simulink library "mbdriLib"  (R2021b)
settings: Solver=ode45  StartTime=0.0  StopTime=10.0  RelTol=1e-3  EnableMultiTasking=on
undefined symbols (not defined in the file or in its folder): ap, deg, DiscIntNeverNeededParam, Earth, env, flat2lla, Newton, rad, Raphson, s, uavData, WGS84, Xpoints, Ypoints, Zpoints
libraries: simulink x23, $bdroot x7, aerolibconvert2 x2, slpidlib x1, sharedtransform x1, SignalEditorBlockLib x1, aerolibtransform2 x1
(part 1 of 2)
settings Model: Creator=mlizarra  LastModifiedBy=promero
settings SolverCC: AlgebraicLoopSolver=TrustRegion
settings DataIOCC: LimitDataPoints=on
settings OptimizationCC: LifeSpan=inf
settings DebuggingCC: AllowSymbolicDim=off  SFUnexpectedBacktrackingDiag=warning  SFNoUnconditionalDefaultTransitionDiag=warning  SFExecutionAtInitializationDiag=none  SFMachineParentedDataDiag=warning  ArithmeticOperatorsInVariantConditions=warning
settings SFSimCC: SimUseLocalCustomCode=off  CustomCodeUndefinedFunction=UseInterfaceOnly
settings RTWCC: RTWUseLocalCustomCode=off
settings CodeAppCC: StateflowObjectComments=on
settings GRTTargetCC: TargetLangStandard=C89/C90 (ANSI)
settings ConfigComp: CovMetricSettings=dw  CovSaveCumulativeToWorkspaceVar=on  CovSaveSingleToWorkspaceVar=on  CovExternalEMLEnable=off

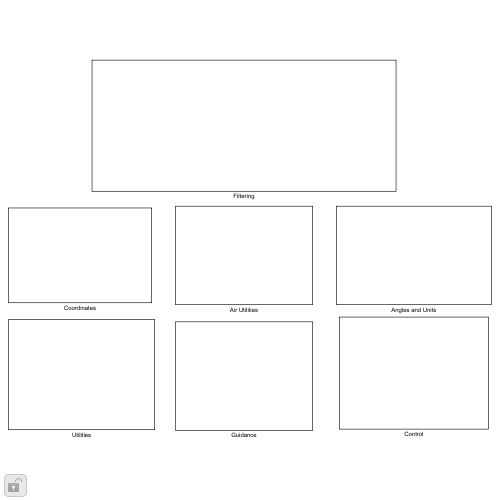
[thumbnail: Simulink's stored preview of the top-level diagram]
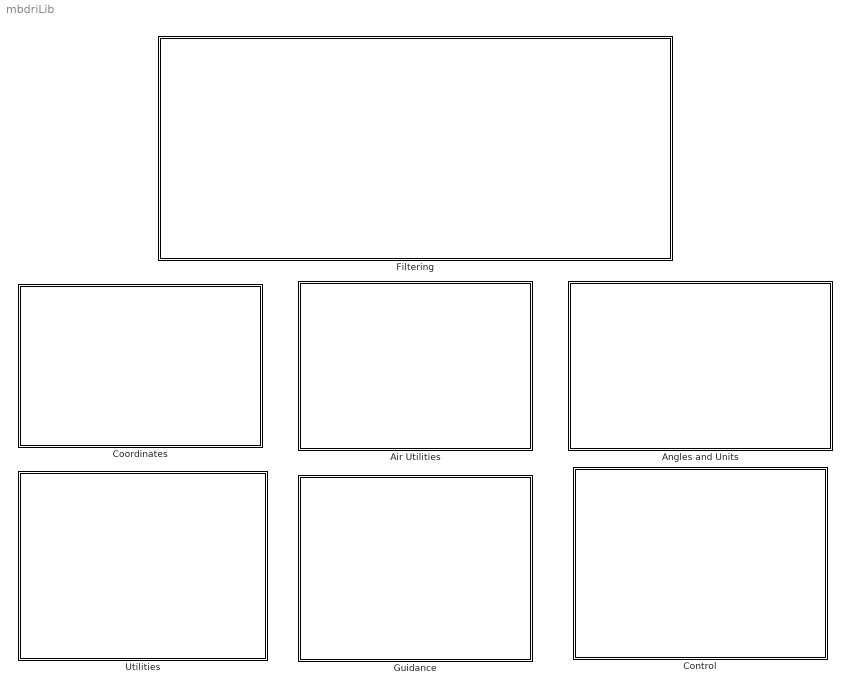
== system mbdriLib ==
  Air Utilities : Subsystem
  Angles and Units : Subsystem
  Control : Subsystem
  Coordinates : Subsystem
  Filtering : Subsystem
  Guidance : Subsystem
  Utilities : Subsystem

== system mbdriLib/Air Utilities ==
  Compute Airspeed : Subsystem

== system mbdriLib/Angles and Units ==
  Lateral Accel to Bank Angle : Subsystem
  psi_dot to phi : Subsystem

== system mbdriLib/Control ==
  PID Controller : Subsystem  mask(PID){Tsample=0.01, Ndelay=5, upperSaturationLimit=100, lowerSaturationLimit=-100}
      mask prompts: Tsample "Sample Time"; Ndelay "Integer delays for de/dt"; upperSaturationLimit "Upper Saturation Limit"; lowerSaturationLimit "Lower Saturation Limit"
      mask help: PID controller block with anti-windup and saturation limits. Implemented as a discrete forwardl integration which stops integrating when the output is saturated. Derivative is implemented as a numerical derivative with N integer delays to smooth output.
      mask Display:
      | disp('PID')
      | port_label('input',1,'error')
      | port_label('input',3,'gains')
      | port_label('input',2,'reset')
      | port_label('output',1,'output')

== system mbdriLib/Coordinates ==
  RL2B : Subsystem

== system mbdriLib/Filtering ==
  1D Discrete Filter : Subsystem  RTWFcnName=TustinFilter3D  mask{bw=40, TSample=0.01}
      mask prompts: bw "Bandwith (Hz)"; TSample "Sample Time"
      mask init:
      | tau = 1/(2*pi*bw);
      | zval = [];
      | pval = -1/tau;
      | kval = 1/tau;
      | 
      | set_param(gcb,'AttributesFormatString', ['Fc = ' num2str(bw)]);
      settings: AttributesFormatString=Fc = 40  RTWFcnNameOpts=User specified  RTWFileNameOpts=Use function name
      mask Display:
      | droots(zval,pval,kval)
      | port_label('input',1,'1D')
  3D Discrete Filter : Subsystem  RTWFcnName=TustinFilter3D  mask{bw=40, TSample=0.01}
      mask prompts: bw "Bandwith (Hz)"; TSample "Sample Time"
      mask init:
      | tau = 1/(2*pi*bw);
      | zval = [];
      | pval = -1/tau;
      | kval = 1/tau;
      | 
      | set_param(gcb,'AttributesFormatString', ['Fc = ' num2str(bw)]);
      settings: AttributesFormatString=Fc = 40  RTWFcnNameOpts=User specified  RTWFileNameOpts=Use function name
      mask Display:
      | droots(zval,pval,kval)
      | port_label('input',1,'3D')
  Complementary Filter : Subsystem  mask{omega=20, T=0.01}
      mask prompts: omega "Cutoff Freq (rad/sec)"; T "Sample Time"
  RateAid for GPS : MATLAB Function  TreatAsAtomicUnit=on
  ZPK 1D Discrete Filter : Subsystem  RTWFcnName=TustinFilter3D  mask{zval=[], pval=[0], kval=1, TSample=0.01}
      mask prompts: zval "Zeros"; pval "Poles"; kval "Gains"; TSample "Sample Time"
      settings: RTWFcnNameOpts=User specified  RTWFileNameOpts=Use function name
      mask Display:
      | droots(zval,pval,kval)
      | port_label('input',1,'1D')
  ZPK 3D Filter : Subsystem  RTWFcnName=TustinFilter3D  mask{zval=[], pval=-1/20, kval=1, TSample=0.01}
      mask prompts: zval "Zeros"; pval "Poles"; kval "Gains"; TSample "Sample Time"
      settings: RTWFcnNameOpts=User specified  RTWFileNameOpts=Use function name
      mask Display:
      | droots(zval,pval,kval)
      | port_label('input',1,'3D')

== system mbdriLib/Guidance ==
  L2+ Guidance Law : Subsystem
  Wp Switching Logic : Stateflow chart  TreatAsAtomicUnit=on

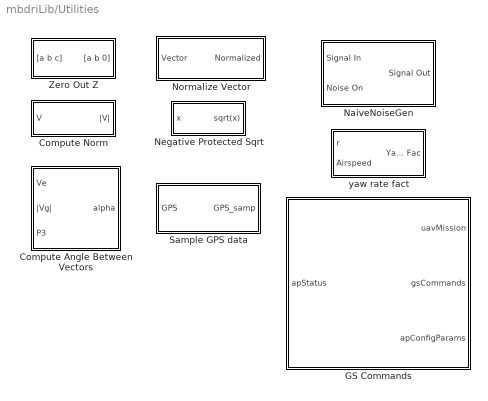
== system mbdriLib/Utilities ==
  " Compute Norm" : Subsystem
  Compute Angle Between Vectors : Subsystem
  "GS Commands " : Subsystem  Variant=on
  NaiveNoiseGen : Subsystem  mask{np=[0.0005], st=ap.apSampleTime, ng=0.2, ns=[1387]}
      mask prompts: np "Noise Power"; st "Sample Time"; ng "Noise Gain"; ns "Noise Seed"
  Negative Protected Sqrt : Subsystem
  Normalize Vector : Subsystem
  Sample GPS data : Subsystem
  Zero Out Z : Subsystem
  yaw rate fact : Subsystem

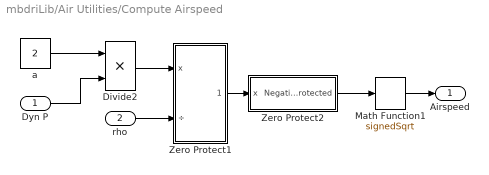
== system mbdriLib/Air Utilities/Compute Airspeed ==
  Dyn P : Inport  Unit=Pa
  rho : Inport  Port=2  Unit=kg/m^3
  Divide2 : Product
  Math Function1 : Sqrt  Operator=signedSqrt  AlgorithmType=Newton-Raphson  SaturateOnIntegerOverflow=on
  Zero Protect1 : Subsystem
      mask Display:
      | disp('Zero\n Protected\nDivision')
      | port_label('input',1,'x')
      | port_label('input',2,'÷')
  Zero Protect2 : Subsystem
      mask Display:
      | disp('Negative\n Protection')
      | port_label('input',1,'u')
      | port_label('output',1,'y')
  a : Constant  Value=2
      settings: AttributesFormatString=%<Value>
  "Airspeed " : Outport  Unit=m/s  VectorParamsAs1DForOutWhenUnconnected=off
  wires:
  Dyn P/1 -> Divide2/2
  a/1 -> Divide2/1
  Zero Protect2/1(Negative Protected) -> Math Function1/1
  Math Function1/1 -> "Airspeed "/1
  Divide2/1 -> Zero Protect1/1(x)
  rho/1 -> Zero Protect1/2(÷)
  Zero Protect1/1(Zero Protected) -> Zero Protect2/1(x)

== system mbdriLib/Angles and Units/Lateral Accel to Bank Angle ==
  a_c : Inport
  Constant : Constant  Value=env.ISA_g
      settings: AttributesFormatString=%<Value>
  Product : Product  Inputs=*/  RndMeth=Zero
  Trigonometric Function : Trigonometry  Operator=atan
  phi_c : Outport  VectorParamsAs1DForOutWhenUnconnected=off
  wires:
  Trigonometric Function/1 -> phi_c/1
  Product/1 -> Trigonometric Function/1
  Constant/1 -> Product/2
  a_c/1 -> Product/1

== system mbdriLib/Angles and Units/psi_dot to phi ==
  psi_dot : Inport  Unit=rad/sec
  U_m : Inport  Port=2  Unit=m/s
  Constant1 : Constant  Value=env.ISA_g
      settings: AttributesFormatString=%<Value>
  Divide : Product  Inputs=**/
  Trigonometric Function : Trigonometry  Operator=atan
  phi : Outport  Unit=rad  VectorParamsAs1DForOutWhenUnconnected=off
  wires:
  psi_dot/1 -> Divide/1
  U_m/1 -> Divide/2
  Constant1/1 -> Divide/3
  Trigonometric Function/1 -> phi/1
  Divide/1 -> Trigonometric Function/1

== system mbdriLib/Control/PID Controller ==
  Error : Inport
  Reset : Inport  Port=2
  PIDGains : Inport  Port=3
  Cast To Boolean : DataTypeConversion  OutDataTypeStr=boolean
  Demux : Demux  Outputs=3
  PID Controller : slpidlib/PID Controller  Controller=PID  Form=Parallel  TimeDomain=Discrete-time  UseExternalTs=off  SampleTime=Tsample  IntegratorMethod=Trapezoidal  FilterMethod=Forward Euler  ControllerParametersSource=external  P=1  I=1  D=0  UseFilter=on  N=100  TunerSelectOption=Transfer Function Based (PID Tuner App)  InitialConditionSource=internal  InitialConditionForIntegrator=0  InitialConditionForFilter=0  DifferentiatorICPrevScaledInput=0  ExternalReset=level  TrackingMode=off  Kt=1  LimitOutput=on  SatLimitsSource=internal  UpperSaturationLimit=upperSaturationLimit  LowerSaturationLimit=lowerSaturationLimit  LinearizeAsGain=on  AntiWindupMode=clamping  Kb=1  POutMin=[]  POutMax=[]  IOutMin=[]  IOutMax=[]  DOutMin=[]  DOutMax=[]  NOutMin=[]  NOutMax=[]  SumOutMin=[]  SumOutMax=[]  SaturationOutMin=[]  SaturationOutMax=[]  PParamMin=[]  PParamMax=[]  IParamMin=[]  IParamMax=[]  DParamMin=[]  DParamMax=[]  NParamMin=[]  NParamMax=[]  KbParamMin=[]  KbParamMax=[]  KtParamMin=[]  KtParamMax=[]  KbOutMin=[]  KbOutMax=[]  KtOutMin=[]  KtOutMax=[]  IntegratorOutMin=[]  IntegratorOutMax=[]  FilterOutMin=[]  FilterOutMax=[]  SumI1OutMin=[]  SumI1OutMax=[]  SumI2OutMin=[]  SumI2OutMax=[]  SumI3OutMin=[]  SumI3OutMax=[]  SumI4OutMin=[]  SumI4OutMax=[]  SumDOutMin=[]  SumDOutMax=[]  DifferentiatorOutMin=[]  DifferentiatorOutMax=[]  FilterDiffOutCoefMin=[]  FilterDiffOutCoefMax=[]  ReciprocalOutMin=[]  ReciprocalOutMax=[]  SumDenOutMin=[]  SumDenOutMax=[]  SumNumOutMin=[]  SumNumOutMax=[]  DivideOutMin=[]  DivideOutMax=[]  UdiffTsProdOutMin=[]  UdiffTsProdOutMax=[]  NTsProdOutMin=[]  NTsProdOutMax=[]  UintegralTsProdOutMin=[]  UintegralTsProdOutMax=[]  UngainTsProdOutMin=[]  UngainTsProdOutMax=[]  IntegratorContinuousStateAttributes=''  IntegratorStateMustResolveToSignalObject=off  IntegratorRTWStateStorageClass=Auto  FilterContinuousStateAttributes=''  FilterStateMustResolveToSignalObject=off  FilterRTWStateStorageClass=Auto  ParallelPVariant=ExternalParameters  IdealPVariant=Disabled  IVariant=ExternalParameters  DVariant=ExternalParameters  IntegratorVariant=Discrete  SatVariant=Enabled  AWVariant=DiscClampingParallel  PCopyVariant=Disabled  TRVariant=Disabled  FdbkBlocksVariant=Feedback  IdealPFdbkVariant=Passthrough  SatFdbkVariant=Passthrough  DerivativeFilterVariant=ForwardEulerFilter  NVariant=ExternalParameters  NCopyVariant=Disabled  FilterICVariant=InternalICsFilter  IntegratorICVariant=InternalICs  ExternalResetVariant=ExternalReset  TRSumVariant=Passthrough  SumFdbkVariant=Enabled  SumVariant=Sum_PID  TsampFilterVariant=InternalTs  TsampNgainVariant=Passthrough  TsampIntegralVariant=Passthrough  ExternalSaturationOutDataTypeStr=Inherit: Same as second input
  delayTime1 : Constant  Value=Ndelay
      settings: AttributesFormatString=%<Value>
  Output : Outport  VectorParamsAs1DForOutWhenUnconnected=off
  wires:
  PIDGains/1 -> Demux/1
  Demux/1 -> PID Controller/2
  Demux/2 -> PID Controller/3
  Demux/3 -> PID Controller/4
  delayTime1/1 -> PID Controller/5
  Reset/1 -> Cast To Boolean/1
  PID Controller/1 -> Output/1
  Error/1 -> PID Controller/1
  Cast To Boolean/1 -> PID Controller/6

== system mbdriLib/Coordinates/RL2B ==
  Euler : Inport
  Rotation Angles to Direction Cosine Matrix : sharedtransform/Rotation Angles to Direction Cosine Matrix  rotationOrder=ZYX  aMode=aMode
      settings: SourceProductBaseCode=AE,PW,DR,MT,UV,VE
  Selector : Selector  InputPortWidth=3  IndexOptions=Index vector (dialog)  Indices=[3 2 1]  OutputSizes=1
  RL2B : Outport  VectorParamsAs1DForOutWhenUnconnected=off
  wires:
  Selector/1 -> Rotation Angles to Direction Cosine Matrix/1
  Euler/1 -> Selector/1
  Rotation Angles to Direction Cosine Matrix/1 -> RL2B/1

== system mbdriLib/Filtering/1D Discrete Filter ==
  In1 : Inport
  Filter4 : Subsystem  mask{Zeros=zval, Poles=pval, Gain=kval, AbsTol=auto, SampleTime=TSample, method=tustin, Wc=1}
      mask prompts: Zeros "Zeros (enter in s-main:)"; Poles "Poles (enter in s-domain:)"; Gain "Gain (enter in s-domain:)"; AbsTol "Absolute tolerance:"; SampleTime "Sample time:"; Wc "Critical Frequency (Hz):"
      mask init:
      | H = zpk(Zeros, Poles, Gain);
      | Hd = c2d(H, SampleTime, 'tustin');
      | [z, p, g] = zpkdata(Hd);
      | z_d = z{:};
      | p_d = p{:};
      | g_d = g;
      mask TypeOptions method: zoh | foh | tustin | prewarp | matched
      mask Display: droots(Zeros,Poles,Gain)
  Out1 : Outport  VectorParamsAs1DForOutWhenUnconnected=off
  wires:
  Filter4/1(Out1) -> Out1/1
  In1/1 -> Filter4/1(In1)

== system mbdriLib/Filtering/3D Discrete Filter ==
  In1 : Inport
  Demux : Demux  Outputs=3
  Filter1 : Subsystem  mask{Zeros=zval, Poles=pval, Gain=kval, AbsTol=auto, SampleTime=TSample, method=tustin, Wc=1}
      mask prompts: Zeros "Zeros (enter in s-main:)"; Poles "Poles (enter in s-domain:)"; Gain "Gain (enter in s-domain:)"; AbsTol "Absolute tolerance:"; SampleTime "Sample time:"; Wc "Critical Frequency (Hz):"
      mask init:
      | H = zpk(Zeros, Poles, Gain);
      | Hd = c2d(H, SampleTime, 'tustin');
      | [z, p, g] = zpkdata(Hd);
      | z_d = z{:};
      | p_d = p{:};
      | g_d = g;
      mask TypeOptions method: zoh | foh | tustin | prewarp | matched
      mask Display: droots(Zeros,Poles,Gain)
  Filter2 : Subsystem  mask{Zeros=zval, Poles=pval, Gain=kval, AbsTol=auto, SampleTime=TSample, method=tustin, Wc=1}
      mask prompts: Zeros "Zeros (enter in s-main:)"; Poles "Poles (enter in s-domain:)"; Gain "Gain (enter in s-domain:)"; AbsTol "Absolute tolerance:"; SampleTime "Sample time:"; Wc "Critical Frequency (Hz):"
      mask init:
      | H = zpk(Zeros, Poles, Gain);
      | Hd = c2d(H, SampleTime, 'tustin');
      | [z, p, g] = zpkdata(Hd);
      | z_d = z{:};
      | p_d = p{:};
      | g_d = g;
      mask TypeOptions method: zoh | foh | tustin | prewarp | matched
      mask Display: droots(Zeros,Poles,Gain)
  Filter4 : Subsystem  mask{Zeros=zval, Poles=pval, Gain=kval, AbsTol=auto, SampleTime=TSample, method=tustin, Wc=1}
      mask prompts: Zeros "Zeros (enter in s-main:)"; Poles "Poles (enter in s-domain:)"; Gain "Gain (enter in s-domain:)"; AbsTol "Absolute tolerance:"; SampleTime "Sample time:"; Wc "Critical Frequency (Hz):"
      mask init:
      | H = zpk(Zeros, Poles, Gain);
      | Hd = c2d(H, SampleTime, 'tustin');
      | [z, p, g] = zpkdata(Hd);
      | z_d = z{:};
      | p_d = p{:};
      | g_d = g;
      mask TypeOptions method: zoh | foh | tustin | prewarp | matched
      mask Display: droots(Zeros,Poles,Gain)
  Mux : Mux  Inputs=3
  Out1 : Outport  VectorParamsAs1DForOutWhenUnconnected=off
  wires:
  Filter2/1(Out1) -> Mux/3
  Filter1/1(Out1) -> Mux/2
  Filter4/1(Out1) -> Mux/1
  Demux/3 -> Filter2/1(In1)
  Demux/2 -> Filter1/1(In1)
  Demux/1 -> Filter4/1(In1)
  In1/1 -> Demux/1
  Mux/1 -> Out1/1

== system mbdriLib/Filtering/Complementary Filter ==
  Rate : Inport
  LoPass : Inport  Port=2
  CutOff : Gain  Gain=omega
      settings: AttributesFormatString=%<Gain>
  Sum : Sum  Inputs=++|
  Sum1 : Sum  Inputs=|+-
  Unit Delay : UnitDelay  SampleTime=ap.apSampleTime  HasFrameUpgradeWarning=on
  ZPK 1D Discrete Filter : $bdroot/Filtering/ZPK 1D Discrete Filter  zval=[]  pval=[0]  kval=1  TSample=ap.apSampleTime
  Blend : Outport  VectorParamsAs1DForOutWhenUnconnected=off
  wires:
  ZPK 1D Discrete Filter/1 -> Blend/1, Unit Delay/1
  Sum/1 -> ZPK 1D Discrete Filter/1  "rate_hat"
  Rate/1 -> Sum/1
  CutOff/1 -> Sum/2
  Sum1/1 -> CutOff/1
  LoPass/1 -> Sum1/1
  Unit Delay/1 -> Sum1/2

== system mbdriLib/Filtering/ZPK 1D Discrete Filter ==
  In1 : Inport
  Filter2 : Subsystem  mask{Zeros=zval, Poles=pval, Gain=kval, AbsTol=auto, SampleTime=TSample, method=tustin, Wc=1}
      mask prompts: Zeros "Zeros (enter in s-main:)"; Poles "Poles (enter in s-domain:)"; Gain "Gain (enter in s-domain:)"; AbsTol "Absolute tolerance:"; SampleTime "Sample time:"; Wc "Critical Frequency (Hz):"
      mask init:
      | H = zpk(Zeros, Poles, Gain);
      | Hd = c2d(H, SampleTime, 'tustin');
      | [z, p, g] = zpkdata(Hd);
      | z_d = z{:};
      | p_d = p{:};
      | g_d = g;
      mask TypeOptions method: zoh | foh | tustin | prewarp | matched
      mask Display: droots(Zeros,Poles,Gain)
  Out1 : Outport  VectorParamsAs1DForOutWhenUnconnected=off
  wires:
  In1/1 -> Filter2/1(In1)
  Filter2/1(Out1) -> Out1/1

== system mbdriLib/Filtering/ZPK 3D Filter ==
  In1 : Inport
  Demux : Demux  Outputs=3
  Filter1 : Subsystem  mask{Zeros=zval, Poles=pval, Gain=kval, AbsTol=auto, SampleTime=TSample, method=tustin, Wc=1}
      mask prompts: Zeros "Zeros (enter in s-main:)"; Poles "Poles (enter in s-domain:)"; Gain "Gain (enter in s-domain:)"; AbsTol "Absolute tolerance:"; SampleTime "Sample time:"; Wc "Critical Frequency (Hz):"
      mask init:
      | H = zpk(Zeros, Poles, Gain);
      | Hd = c2d(H, SampleTime, 'tustin');
      | [z, p, g] = zpkdata(Hd);
      | z_d = z{:};
      | p_d = p{:};
      | g_d = g;
      mask TypeOptions method: zoh | foh | tustin | prewarp | matched
      mask Display: droots(Zeros,Poles,Gain)
  Filter2 : Subsystem  mask{Zeros=zval, Poles=pval, Gain=kval, AbsTol=auto, SampleTime=TSample, method=tustin, Wc=1}
      mask prompts: Zeros "Zeros (enter in s-main:)"; Poles "Poles (enter in s-domain:)"; Gain "Gain (enter in s-domain:)"; AbsTol "Absolute tolerance:"; SampleTime "Sample time:"; Wc "Critical Frequency (Hz):"
      mask init:
      | H = zpk(Zeros, Poles, Gain);
      | Hd = c2d(H, SampleTime, 'tustin');
      | [z, p, g] = zpkdata(Hd);
      | z_d = z{:};
      | p_d = p{:};
      | g_d = g;
      mask TypeOptions method: zoh | foh | tustin | prewarp | matched
      mask Display: droots(Zeros,Poles,Gain)
  Filter4 : Subsystem  mask{Zeros=zval, Poles=pval, Gain=kval, AbsTol=auto, SampleTime=TSample, method=tustin, Wc=1}
      mask prompts: Zeros "Zeros (enter in s-main:)"; Poles "Poles (enter in s-domain:)"; Gain "Gain (enter in s-domain:)"; AbsTol "Absolute tolerance:"; SampleTime "Sample time:"; Wc "Critical Frequency (Hz):"
      mask init:
      | H = zpk(Zeros, Poles, Gain);
      | Hd = c2d(H, SampleTime, 'tustin');
      | [z, p, g] = zpkdata(Hd);
      | z_d = z{:};
      | p_d = p{:};
      | g_d = g;
      mask TypeOptions method: zoh | foh | tustin | prewarp | matched
      mask Display: droots(Zeros,Poles,Gain)
  Mux : Mux  Inputs=3
  Out1 : Outport  VectorParamsAs1DForOutWhenUnconnected=off
  wires:
  Mux/1 -> Out1/1
  In1/1 -> Demux/1
  Demux/1 -> Filter4/1(In1)
  Demux/2 -> Filter1/1(In1)
  Demux/3 -> Filter2/1(In1)
  Filter4/1(Out1) -> Mux/1
  Filter1/1(Out1) -> Mux/2
  Filter2/1(Out1) -> Mux/3

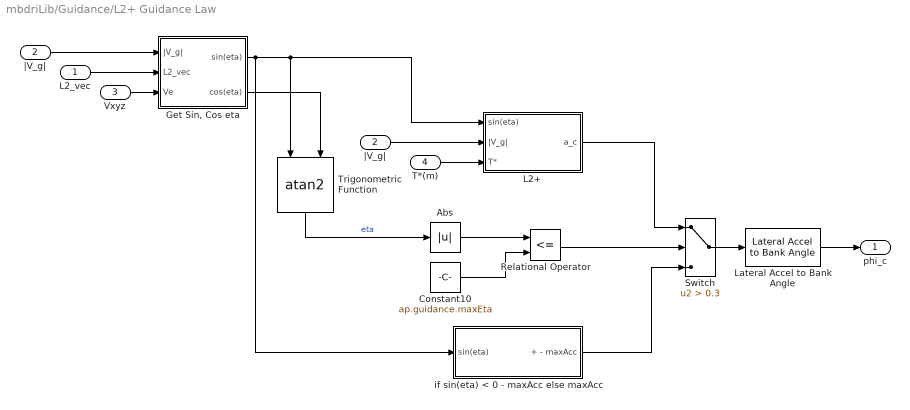
== system mbdriLib/Guidance/L2+ Guidance Law ==
  L2_vec : Inport
  |V_g| : Inport  Port=2  Unit=m/s
  Vxyz : Inport  Port=3  Unit=m/s
  T*(m) : Inport  Port=4  Unit=m
  Abs : Abs
  Constant10 : Constant  Value=ap.guidance.maxEta
      settings: AttributesFormatString=%<Value>
  "Get Sin, Cos eta" : Subsystem
  L2+ : Subsystem
  Lateral Accel to Bank Angle : $bdroot/Angles and Units/Lateral Accel to  Bank Angle  SystemSampleTime=-1  VariantActivationTime=update diagram  Latency=0  AutoFrameSizeCalculation=off
  Relational Operator : RelationalOperator  Operator=<=  OutDataTypeStr=boolean  RndMeth=Nearest
  Switch : Switch  Criteria=u2 > Threshold  Threshold=0.3
  Trigonometric Function : Trigonometry  Operator=atan2
  "if sin(eta) < 0 - maxAcc else maxAcc " : Subsystem
  "|V_g| " : InportShadow  Port=2  Unit=m/s
  phi_c : Outport  Unit=rad  VectorParamsAs1DForOutWhenUnconnected=off
  wires:
  "Get Sin, Cos eta"/2(cos(eta)) -> Trigonometric Function/2
  L2+/1(a_c) -> Switch/1
  Lateral Accel to Bank Angle/1 -> phi_c/1
  T*(m)/1 -> L2+/3(T*)
  "|V_g| "/1 -> L2+/2(|V_g|)
  "Get Sin, Cos eta"/1(sin(eta)) -> Trigonometric Function/1, L2+/1(sin(eta)), "if sin(eta) < 0 - maxAcc else maxAcc "/1(sin(eta))
  Trigonometric Function/1 -> Abs/1  "eta"
  Abs/1 -> Relational Operator/1
  Constant10/1 -> Relational Operator/2
  Relational Operator/1 -> Switch/2
  "if sin(eta) < 0 - maxAcc else maxAcc "/1(+ - maxAcc) -> Switch/3
  Switch/1 -> Lateral Accel to Bank Angle/1
  |V_g|/1 -> "Get Sin, Cos eta"/1(|V_g|)
  L2_vec/1 -> "Get Sin, Cos eta"/2(L2_vec)
  Vxyz/1 -> "Get Sin, Cos eta"/3(Ve)

== system mbdriLib/Utilities/ Compute Norm ==
  V : Inport
  Dot Product : DotProduct  InputSameDT=on  OutDataTypeStr=Inherit: Inherit via internal rule
  Negative Protected Sqrt : $bdroot/Utilities/Negative Protected Sqrt  SystemSampleTime=-1  VariantActivationTime=update diagram  Latency=0  AutoFrameSizeCalculation=off
  |V| : Outport  VectorParamsAs1DForOutWhenUnconnected=off
  wires:
  Dot Product/1 -> Negative Protected Sqrt/1
  V/1 -> Dot Product/1, Dot Product/2
  Negative Protected Sqrt/1 -> |V|/1

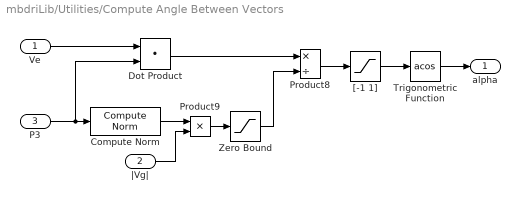
== system mbdriLib/Utilities/Compute Angle Between Vectors ==
  Ve : Inport
  |Vg| : Inport  Port=2
  P3 : Inport  Port=3
  " Compute Norm" : $bdroot/Utilities/ Compute Norm  SystemSampleTime=-1  VariantActivationTime=update diagram  Latency=0  AutoFrameSizeCalculation=off
  Dot Product : DotProduct  InputSameDT=on  OutDataTypeStr=Inherit: Inherit via internal rule
  Product8 : Product  Inputs=*/  RndMeth=Zero
  Product9 : Product  RndMeth=Zero
  Trigonometric Function : Trigonometry  Operator=acos
  Zero Bound : Saturate  UpperLimit=inf  LowerLimit=0.001
      settings: AttributesFormatString="[%<LowerLimit>  %<UpperLimit>]"
  "[-1 1]" : Saturate  UpperLimit=1  LowerLimit=-1
      settings: AttributesFormatString="[%<LowerLimit>  %<UpperLimit>]"
  alpha : Outport  VectorParamsAs1DForOutWhenUnconnected=off
  wires:
  P3/1 -> " Compute Norm"/1, Dot Product/2
  Ve/1 -> Dot Product/1
  Dot Product/1 -> Product8/1
  " Compute Norm"/1 -> Product9/1
  |Vg|/1 -> Product9/2
  Product9/1 -> Zero Bound/1
  Product8/1 -> "[-1 1]"/1
  "[-1 1]"/1 -> Trigonometric Function/1
  Zero Bound/1 -> Product8/2
  Trigonometric Function/1 -> alpha/1

== system mbdriLib/Utilities/GS Commands  ==
  apStatus : Inport  OutDataTypeStr=Bus: apStatusBus
  Use QGroundControl : Subsystem  VariantControl=useQGCvar
  Use Simulink : Subsystem  VariantControl=useSLvar
  uavMission : Outport  OutDataTypeStr=Bus: waypoint  VectorParamsAs1DForOutWhenUnconnected=off
  gsCommands : Outport  Port=2  OutDataTypeStr=Bus: gsCommandsBus  VectorParamsAs1DForOutWhenUnconnected=off
  apConfigParams : Outport  Port=3  OutDataTypeStr=Bus: apConfigParamsBus  VectorParamsAs1DForOutWhenUnconnected=off

== system mbdriLib/Utilities/NaiveNoiseGen ==
  Signal In : Inport
  Noise On : Inport  Port=2
  Add : Sum
  Band-Limited White Noise : simulink/Sources/Band-Limited White Noise  Cov=np  Ts=st  seed=ns
  Gain : Gain  Gain=ng
      settings: AttributesFormatString=%<Gain>
  Switch : Switch  Threshold=0.3
  Signal Out : Outport  VectorParamsAs1DForOutWhenUnconnected=off
  wires:
  Band-Limited White Noise/1 -> Gain/1
  Add/1 -> Switch/1
  Noise On/1 -> Switch/2
  Switch/1 -> Signal Out/1
  Signal In/1 -> Switch/3, Add/1
  Gain/1 -> Add/2

== system mbdriLib/Utilities/Negative Protected Sqrt ==
  x : Inport
  Math Function1 : Sqrt  OutputSignalType=real  AlgorithmType=Newton-Raphson  SaturateOnIntegerOverflow=on
      settings: AttributesFormatString=%<AlgorithmType>
  Zero Bound : Saturate  UpperLimit=inf  LowerLimit=0.001
      settings: AttributesFormatString="[%<LowerLimit>  %<UpperLimit>]"
  sqrt(x) : Outport  VectorParamsAs1DForOutWhenUnconnected=off
  wires:
  x/1 -> Zero Bound/1
  Math Function1/1 -> sqrt(x)/1
  Zero Bound/1 -> Math Function1/1

== system mbdriLib/Utilities/Normalize Vector ==
  Vector : Inport
  " Compute Norm" : $bdroot/Utilities/ Compute Norm  SystemSampleTime=-1  VariantActivationTime=update diagram  Latency=0  AutoFrameSizeCalculation=off
  Divide : Product  Inputs=*/
  Normalized : Outport  VectorParamsAs1DForOutWhenUnconnected=off
  wires:
  Vector/1 -> Divide/1, " Compute Norm"/1
  " Compute Norm"/1 -> Divide/2
  Divide/1 -> Normalized/1

== system mbdriLib/Utilities/Sample GPS data ==
  GPS : Inport
  Rate Transition : RateTransition  Deterministic=off  OutPortSampleTime=sensors.gpsRefreshRate
      settings: AttributesFormatString=%<OutPortSampleTime>
  GPS_samp : Outport  VectorParamsAs1DForOutWhenUnconnected=off
  wires:
  GPS/1 -> Rate Transition/1
  Rate Transition/1 -> GPS_samp/1

== system mbdriLib/Utilities/Zero Out Z ==
  "[a b c]" : Inport
  Constant : Constant  Value=0
      settings: AttributesFormatString=%<Value>
  Demux : Demux  Outputs=[2 1]
  Mux : Mux  Inputs=2
  Terminator : Terminator
  "[a b 0]" : Outport  VectorParamsAs1DForOutWhenUnconnected=off
  wires:
  "[a b c]"/1 -> Demux/1
  Constant/1 -> Mux/2
  Demux/2 -> Terminator/1
  Mux/1 -> "[a b 0]"/1
  Demux/1 -> Mux/1

== system mbdriLib/Utilities/yaw rate fact ==
  r : Inport
  Airspeed : Inport  Port=2
  Cmq3 : Constant  Value=.5
      settings: AttributesFormatString=%<Value>
  Cmq4 : Constant  Value=uavData.geometry.span
      settings: AttributesFormatString=%<Value>
  Product1 : Product  Inputs=***/  SaturateOnIntegerOverflow=on  OutDataTypeStr=Inherit: Same as first input
  Saturation : Saturate  UpperLimit=inf  LowerLimit=0.1
      settings: AttributesFormatString="[%<LowerLimit>  %<UpperLimit>]"
  Yaw Rate Fac : Outport  VectorParamsAs1DForOutWhenUnconnected=off
  wires:
  Saturation/1 -> Product1/4
  Airspeed/1 -> Saturation/1
  Cmq4/1 -> Product1/3
  Cmq3/1 -> Product1/2
  r/1 -> Product1/1
  Product1/1 -> Yaw Rate Fac/1

== system mbdriLib/Air Utilities/Compute Airspeed/Zero Protect1 ==
  x : Inport
  ÷ : Inport  Port=2
  Divide2 : Product  Inputs=*/
  Switch : Switch  Criteria=u2 ~= 0  Threshold=0.1  OutDataTypeStr=Inherit: Inherit via back propagation
  Zero Value : Constant  Value=0
  Zero Protected : Outport  VectorParamsAs1DForOutWhenUnconnected=off
  wires:
  ÷/1 -> Switch/2, Divide2/2
  Zero Value/1 -> Switch/3
  Switch/1 -> Zero Protected/1
  Divide2/1 -> Switch/1
  x/1 -> Divide2/1

== system mbdriLib/Air Utilities/Compute Airspeed/Zero Protect2 ==
  x : Inport
  Switch : Switch  OutDataTypeStr=Inherit: Inherit via back propagation
  Zero Value : Constant  Value=0
  Negative Protected : Outport  VectorParamsAs1DForOutWhenUnconnected=off
  wires:
  x/1 -> Switch/2, Switch/1
  Switch/1 -> Negative Protected/1
  Zero Value/1 -> Switch/3

== system mbdriLib/Filtering/1D Discrete Filter/Filter4 ==
  In1 : Inport
  Discrete Zero-Pole : DiscreteZeroPole  Zeros=z_d  Poles=p_d  Gain=g_d  SampleTime=-1
  Out1 : Outport  VectorParamsAs1DForOutWhenUnconnected=off
  wires:
  Discrete Zero-Pole/1 -> Out1/1
  In1/1 -> Discrete Zero-Pole/1

== system mbdriLib/Filtering/3D Discrete Filter/Filter1 ==
  In1 : Inport
  Discrete Zero-Pole : DiscreteZeroPole  Zeros=z_d  Poles=p_d  Gain=g_d  SampleTime=-1
  Out1 : Outport  VectorParamsAs1DForOutWhenUnconnected=off
  wires:
  Discrete Zero-Pole/1 -> Out1/1
  In1/1 -> Discrete Zero-Pole/1

== system mbdriLib/Filtering/3D Discrete Filter/Filter2 ==
  In1 : Inport
  Discrete Zero-Pole : DiscreteZeroPole  Zeros=z_d  Poles=p_d  Gain=g_d  SampleTime=-1
  Out1 : Outport  VectorParamsAs1DForOutWhenUnconnected=off
  wires:
  In1/1 -> Discrete Zero-Pole/1
  Discrete Zero-Pole/1 -> Out1/1

== system mbdriLib/Filtering/3D Discrete Filter/Filter4 ==
  In1 : Inport
  Discrete Zero-Pole : DiscreteZeroPole  Zeros=z_d  Poles=p_d  Gain=g_d  SampleTime=-1
  Out1 : Outport  VectorParamsAs1DForOutWhenUnconnected=off
  wires:
  In1/1 -> Discrete Zero-Pole/1
  Discrete Zero-Pole/1 -> Out1/1

== system mbdriLib/Filtering/ZPK 1D Discrete Filter/Filter2 ==
  In1 : Inport
  Discrete Zero-Pole : DiscreteZeroPole  Zeros=z_d  Poles=p_d  Gain=g_d  SampleTime=-1
  Out1 : Outport  VectorParamsAs1DForOutWhenUnconnected=off
  wires:
  In1/1 -> Discrete Zero-Pole/1
  Discrete Zero-Pole/1 -> Out1/1

== system mbdriLib/Filtering/ZPK 3D Filter/Filter1 ==
  In1 : Inport
  Discrete Zero-Pole : DiscreteZeroPole  Zeros=z_d  Poles=p_d  Gain=g_d  SampleTime=-1
  Out1 : Outport  VectorParamsAs1DForOutWhenUnconnected=off
  wires:
  In1/1 -> Discrete Zero-Pole/1
  Discrete Zero-Pole/1 -> Out1/1

== system mbdriLib/Filtering/ZPK 3D Filter/Filter2 ==
  In1 : Inport
  Discrete Zero-Pole : DiscreteZeroPole  Zeros=z_d  Poles=p_d  Gain=g_d  SampleTime=-1
  Out1 : Outport  VectorParamsAs1DForOutWhenUnconnected=off
  wires:
  Discrete Zero-Pole/1 -> Out1/1
  In1/1 -> Discrete Zero-Pole/1

== system mbdriLib/Filtering/ZPK 3D Filter/Filter4 ==
  In1 : Inport
  Discrete Zero-Pole : DiscreteZeroPole  Zeros=z_d  Poles=p_d  Gain=g_d  SampleTime=-1
  Out1 : Outport  VectorParamsAs1DForOutWhenUnconnected=off
  wires:
  Discrete Zero-Pole/1 -> Out1/1
  In1/1 -> Discrete Zero-Pole/1

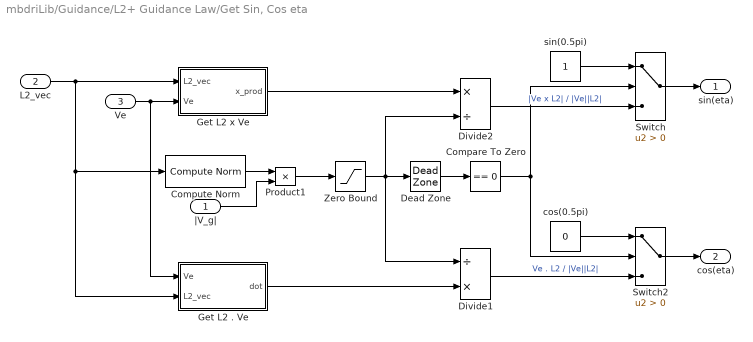
== system mbdriLib/Guidance/L2+ Guidance Law/Get Sin, Cos eta ==
  |V_g| : Inport
  L2_vec : Inport  Port=2
  Ve : Inport  Port=3
  " Compute Norm" : $bdroot/Utilities/ Compute Norm  SystemSampleTime=-1  VariantActivationTime=update diagram  Latency=0  AutoFrameSizeCalculation=off
  Compare To Zero : simulink/Logic and Bit Operations/Compare To Zero  relop===  OutDataTypeStr=boolean  ZeroCross=off
  Dead Zone : DeadZone  LowerValue=-0.1  UpperValue=0.1  SaturateOnIntegerOverflow=on
  Divide1 : Product  Inputs=/*
  Divide2 : Product  Inputs=*/
  Get L2 . Ve : Subsystem
  Get L2 x Ve : Subsystem
  Product1 : Product  RndMeth=Zero
  Switch : Switch  Criteria=u2 > Threshold  ZeroCross=off
  Switch2 : Switch  Criteria=u2 > Threshold  ZeroCross=off
  Zero Bound : Saturate  UpperLimit=inf  LowerLimit=0.001
      settings: AttributesFormatString="[%<LowerLimit>  %<UpperLimit>]"
  cos(0.5pi) : Constant  Value=0
      settings: AttributesFormatString=%<Value>
  sin(0.5pi) : Constant
      settings: AttributesFormatString=%<Value>
  sin(eta) : Outport  VectorParamsAs1DForOutWhenUnconnected=off
  cos(eta) : Outport  Port=2  VectorParamsAs1DForOutWhenUnconnected=off
  wires:
  Compare To Zero/1 -> Switch/2, Switch2/2
  Dead Zone/1 -> Compare To Zero/1
  L2_vec/1 -> Get L2 x Ve/1(L2_vec), Get L2 . Ve/2(L2_vec), " Compute Norm"/1
  Ve/1 -> Get L2 x Ve/2(Ve), Get L2 . Ve/1(Ve)
  " Compute Norm"/1 -> Product1/1
  |V_g|/1 -> Product1/2
  Product1/1 -> Zero Bound/1
  Get L2 . Ve/1(dot) -> Divide1/2
  sin(0.5pi)/1 -> Switch/1
  Switch2/1 -> cos(eta)/1
  cos(0.5pi)/1 -> Switch2/1
  Divide1/1 -> Switch2/3  "Ve . L2 / |Ve||L2|"
  Get L2 x Ve/1(x_prod) -> Divide2/1
  Divide2/1 -> Switch/3  "|Ve x L2| / |Ve||L2|"
  Switch/1 -> sin(eta)/1
  Zero Bound/1 -> Dead Zone/1, Divide2/2, Divide1/1

== system mbdriLib/Guidance/L2+ Guidance Law/L2+ ==
  sin(eta) : Inport
  |V_g| : Inport  Port=2
  T* : Inport  Port=3
  Divide : Product  Inputs=**/
  Gain : Gain  Gain=2
      settings: AttributesFormatString=%<Gain>
  Zero Bound : Saturate  UpperLimit=inf  LowerLimit=0.001
      settings: AttributesFormatString="[%<LowerLimit>  %<UpperLimit>]"
  a_c : Outport  VectorParamsAs1DForOutWhenUnconnected=off
  wires:
  Zero Bound/1 -> Divide/3
  sin(eta)/1 -> Divide/1
  Divide/1 -> Gain/1
  |V_g|/1 -> Divide/2
  Gain/1 -> a_c/1
  T*/1 -> Zero Bound/1

== system mbdriLib/Guidance/L2+ Guidance Law/if sin(eta) < 0 - maxAcc else maxAcc  ==
  sin(eta) : Inport
  Compare To Zero : simulink/Logic and Bit Operations/Compare To Zero  relop=<  OutDataTypeStr=boolean  ZeroCross=off
  Constant1 : Constant  Value=ap.guidance.maxAcc
      settings: AttributesFormatString=%<Value>
  Constant9 : Constant  Value=-ap.guidance.maxAcc
      settings: AttributesFormatString=%<Value>
  Switch1 : Switch  Criteria=u2 ~= 0  Threshold=0.3
  + - maxAcc : Outport  VectorParamsAs1DForOutWhenUnconnected=off
  wires:
  Compare To Zero/1 -> Switch1/2
  Constant9/1 -> Switch1/1
  Constant1/1 -> Switch1/3
  sin(eta)/1 -> Compare To Zero/1
  Switch1/1 -> + - maxAcc/1

== system mbdriLib/Utilities/GS Commands /Use QGroundControl ==
  apStatus : Inport  OutDataTypeStr=Bus: apStatusBus
  Send to QGC : ModelReference  ModelNameDialog=QGroundControlInterface  ModelReferenceVersion=1.374
  uavMission : Outport  OutDataTypeStr=Bus: waypoint  VectorParamsAs1DForOutWhenUnconnected=off
  gsCommands : Outport  Port=2  OutDataTypeStr=Bus: gsCommandsBus  VectorParamsAs1DForOutWhenUnconnected=off
  apConfigParams : Outport  Port=3  OutDataTypeStr=Bus: apConfigParamsBus  VectorParamsAs1DForOutWhenUnconnected=off
  wires:
  Send to QGC/1 -> uavMission/1
  Send to QGC/2 -> apConfigParams/1
  apStatus/1 -> Send to QGC/1
  Send to QGC/3 -> gsCommands/1

== system mbdriLib/Utilities/GS Commands /Use Simulink ==
  apStatus : Inport  OutDataTypeStr=Bus: apStatusBus
  AP Config Parameters : Subsystem
  Ground Station Commands : Subsystem
  Terminator : Terminator
  Waypoint Mission : Subsystem
  uavMission : Outport  OutDataTypeStr=Bus: waypoint  VectorParamsAs1DForOutWhenUnconnected=off
  gsCommands : Outport  Port=2  OutDataTypeStr=Bus: gsCommandsBus  VectorParamsAs1DForOutWhenUnconnected=off
  apConfigParams : Outport  Port=3  OutDataTypeStr=Bus: apConfigParamsBus  VectorParamsAs1DForOutWhenUnconnected=off
  wires:
  Waypoint Mission/1(uavMission) -> uavMission/1
  AP Config Parameters/1(apConfigParams) -> apConfigParams/1
  apStatus/1 -> Terminator/1
  Ground Station Commands/1(gsCommands) -> gsCommands/1

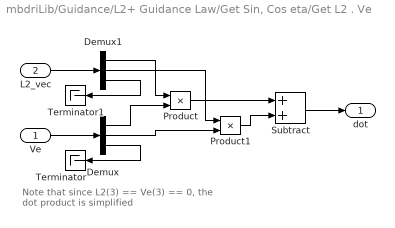
== system mbdriLib/Guidance/L2+ Guidance Law/Get Sin, Cos eta/Get L2 . Ve ==
  note: Note that since L2(3) == Ve(3) == 0, the
      | dot product is simplified
  Ve : Inport
  L2_vec : Inport  Port=2
  Demux : Demux  Outputs=3
  Demux1 : Demux  Outputs=3
  Product : Product  RndMeth=Zero
  Product1 : Product  RndMeth=Zero
  Subtract : Sum  Inputs=2
  Terminator : Terminator
  Terminator1 : Terminator
  dot : Outport  VectorParamsAs1DForOutWhenUnconnected=off
  wires:
  Ve/1 -> Demux/1
  Subtract/1 -> dot/1
  L2_vec/1 -> Demux1/1
  Product1/1 -> Subtract/2
  Product/1 -> Subtract/1
  Demux1/3 -> Terminator1/1
  Demux/3 -> Terminator/1
  Demux1/1 -> Product/1
  Demux/1 -> Product/2
  Demux1/2 -> Product1/1
  Demux/2 -> Product1/2

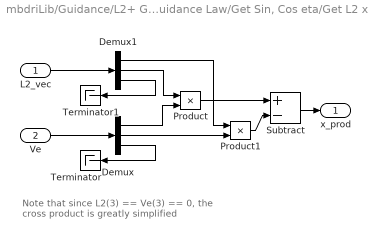
== system mbdriLib/Guidance/L2+ Guidance Law/Get Sin, Cos eta/Get L2 x Ve ==
  note: Note that since L2(3) == Ve(3) == 0, the
      | cross product is greatly simplified
  L2_vec : Inport
  Ve : Inport  Port=2
  Demux : Demux  Outputs=3
  Demux1 : Demux  Outputs=3
  Product : Product  RndMeth=Zero
  Product1 : Product  RndMeth=Zero
  Subtract : Sum  Inputs=+-
  Terminator : Terminator
  Terminator1 : Terminator
  x_prod : Outport  VectorParamsAs1DForOutWhenUnconnected=off
  wires:
  Demux/3 -> Terminator/1
  Demux1/3 -> Terminator1/1
  Demux/1 -> Product/2
  Demux1/2 -> Product/1
  Demux/2 -> Product1/2
  Demux1/1 -> Product1/1
  Product/1 -> Subtract/1
  Product1/1 -> Subtract/2
  L2_vec/1 -> Demux1/1
  Subtract/1 -> x_prod/1
  Ve/1 -> Demux/1

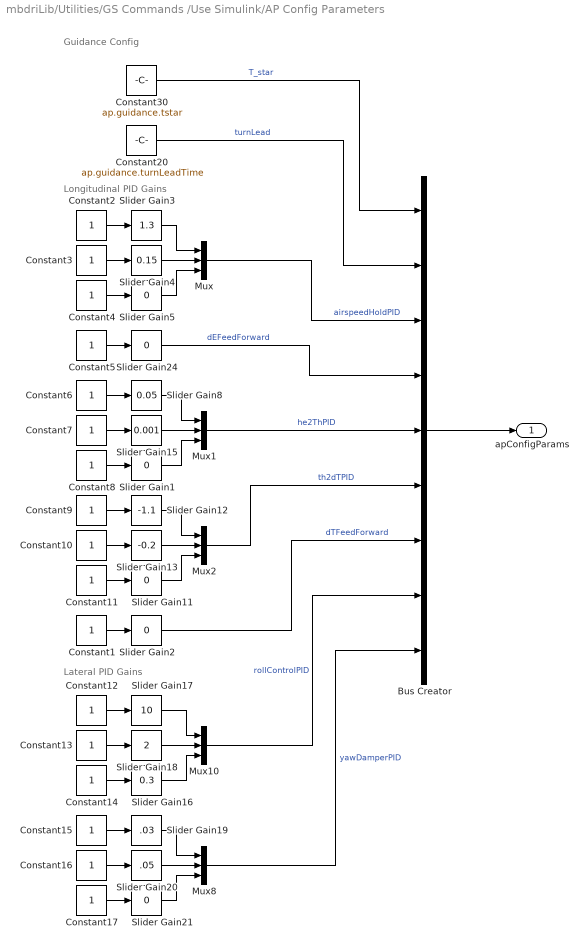
== system mbdriLib/Utilities/GS Commands /Use Simulink/AP Config Parameters ==
  note: Guidance Config
  note: Lateral PID Gains
  note: Longitudinal PID Gains
  Bus Creator : BusCreator  Inputs=9  OutDataTypeStr=Bus: apConfigParamsBus
  Constant{1..17} (17 alike) : Constant  SampleTime=ap.apSampleTime
      settings: AttributesFormatString=%<Value>
  Constant20 : Constant  Value=ap.guidance.turnLeadTime  SampleTime=ap.apSampleTime
      settings: AttributesFormatString=%<Value>
  Constant30 : Constant  Value=ap.guidance.tstar  SampleTime=ap.apSampleTime
      settings: AttributesFormatString=%<Value>
  Mux{,1..2,8,10} (5 alike) : Mux  Inputs=3
  Slider Gain1 : simulink/Math Operations/Slider Gain  gain=0  low=-20  high=20
  Slider Gain11 : simulink/Math Operations/Slider Gain  gain=0  low=-0.1  high=0
  Slider Gain12 : simulink/Math Operations/Slider Gain  gain=-1.1  low=-2  high=0.5
  Slider Gain13 : simulink/Math Operations/Slider Gain  gain=-0.2  low=-0.2  high=0
  Slider Gain15 : simulink/Math Operations/Slider Gain  gain=0.001  low=-20  high=20
  Slider Gain16 : simulink/Math Operations/Slider Gain  gain=0.3  low=-0.1  high=5
  Slider Gain17 : simulink/Math Operations/Slider Gain  gain=10  low=-0.1  high=50
  Slider Gain18 : simulink/Math Operations/Slider Gain  gain=2  low=0  high=2
  Slider Gain19 : simulink/Math Operations/Slider Gain  gain=.03  low=-20  high=20
  Slider Gain2 : simulink/Math Operations/Slider Gain  gain=0  low=-0.1  high=5
  Slider Gain20 : simulink/Math Operations/Slider Gain  gain=.05  low=-20  high=20
  Slider Gain21 : simulink/Math Operations/Slider Gain  gain=0  low=-20  high=20
  Slider Gain24 : simulink/Math Operations/Slider Gain  gain=0  low=-0.1  high=5
  Slider Gain3 : simulink/Math Operations/Slider Gain  gain=1.3  low=-0.5  high=4.5
  Slider Gain4 : simulink/Math Operations/Slider Gain  gain=0.15  low=-20  high=20
  Slider Gain5 : simulink/Math Operations/Slider Gain  gain=0  low=-20  high=20
  Slider Gain8 : simulink/Math Operations/Slider Gain  gain=0.05  low=-20  high=20
  apConfigParams : Outport  OutDataTypeStr=Bus: apConfigParamsBus  VectorParamsAs1DForOutWhenUnconnected=off
  wires:
  Bus Creator/1 -> apConfigParams/1
  Constant30/1 -> Bus Creator/1  "T_star"
  Constant20/1 -> Bus Creator/2  "turnLead"
  Constant2/1 -> Slider Gain3/1
  Constant3/1 -> Slider Gain4/1
  Constant4/1 -> Slider Gain5/1
  Slider Gain4/1 -> Mux/2
  Slider Gain3/1 -> Mux/1
  Slider Gain5/1 -> Mux/3
  Mux/1 -> Bus Creator/3  "airspeedHoldPID"
  Constant5/1 -> Slider Gain24/1
  Slider Gain24/1 -> Bus Creator/4  "dEFeedForward"
  Constant6/1 -> Slider Gain8/1
  Constant7/1 -> Slider Gain15/1
  Constant8/1 -> Slider Gain1/1
  Slider Gain8/1 -> Mux1/1
  Mux1/1 -> Bus Creator/5  "he2ThPID"
  Constant9/1 -> Slider Gain12/1
  Constant10/1 -> Slider Gain13/1
  Constant11/1 -> Slider Gain11/1
  Slider Gain13/1 -> Mux2/2
  Slider Gain12/1 -> Mux2/1
  Slider Gain11/1 -> Mux2/3
  Mux2/1 -> Bus Creator/6  "th2dTPID"
  Slider Gain15/1 -> Mux1/2
  Slider Gain1/1 -> Mux1/3
  Constant1/1 -> Slider Gain2/1
  Slider Gain2/1 -> Bus Creator/7  "dTFeedForward"
  Constant12/1 -> Slider Gain17/1
  Constant13/1 -> Slider Gain18/1
  Constant14/1 -> Slider Gain16/1
  Slider Gain18/1 -> Mux10/2
  Slider Gain17/1 -> Mux10/1
  Slider Gain16/1 -> Mux10/3
  Mux10/1 -> Bus Creator/8  "rollControlPID"
  Constant15/1 -> Slider Gain19/1
  Constant16/1 -> Slider Gain20/1
  Constant17/1 -> Slider Gain21/1
  Slider Gain20/1 -> Mux8/2
  Slider Gain19/1 -> Mux8/1
  Slider Gain21/1 -> Mux8/3
  Mux8/1 -> Bus Creator/9  "yawDamperPID"

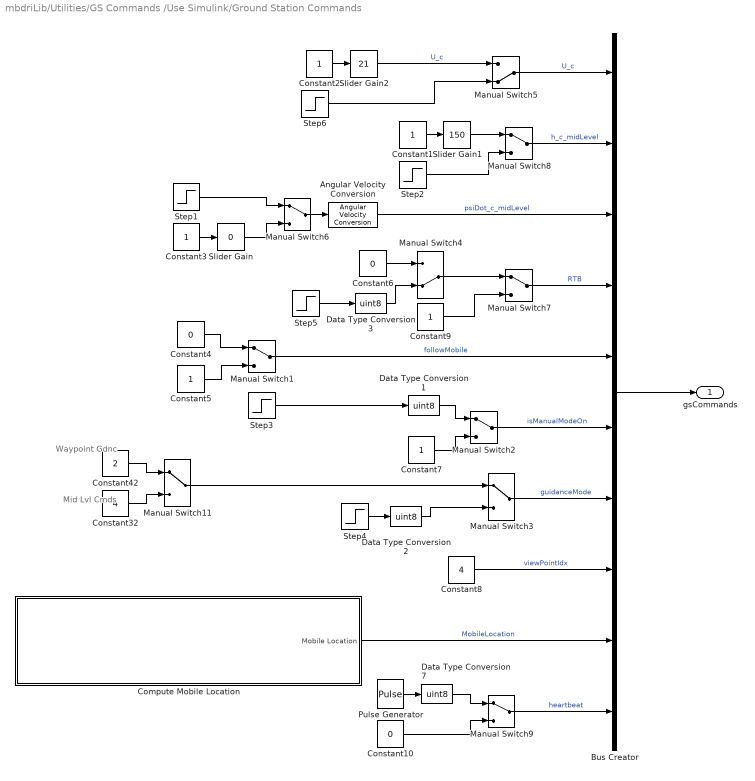
== system mbdriLib/Utilities/GS Commands /Use Simulink/Ground Station Commands ==
  note: Mid Lvl
      | Cmds
  note: Waypoint
      | Gdnc
  Angular Velocity Conversion : aerolibconvert2/Angular Velocity Conversion  IU=deg/s  OU=rad/s
  Bus Creator : BusCreator  Inputs=10  OutDataTypeStr=Bus: gsCommandsBus  NonVirtualBus=on
  Compute Mobile Location : Subsystem
  Constant1 : Constant  OutDataTypeStr=single  SampleTime=ap.apSampleTime
      settings: AttributesFormatString=%<Value>
  Constant10 : Constant  Value=0  OutDataTypeStr=uint8  SampleTime=ap.apSampleTime
      settings: AttributesFormatString=%<Value>
  Constant2 : Constant  SampleTime=ap.apSampleTime
      settings: AttributesFormatString=%<Value>
  Constant3 : Constant  SampleTime=ap.apSampleTime
      settings: AttributesFormatString=%<Value>
  Constant32 : Constant  Value=4  OutDataTypeStr=uint8  SampleTime=ap.apSampleTime
      settings: AttributesFormatString=%<Value>
  Constant4 : Constant  Value=0  OutDataTypeStr=uint8  SampleTime=ap.apSampleTime
      settings: AttributesFormatString=%<Value>
  Constant42 : Constant  Value=2  OutDataTypeStr=uint8  SampleTime=ap.apSampleTime
      settings: AttributesFormatString=%<Value>
  Constant5 : Constant  OutDataTypeStr=uint8  SampleTime=ap.apSampleTime
      settings: AttributesFormatString=%<Value>
  Constant6 : Constant  Value=0  OutDataTypeStr=uint8  SampleTime=ap.apSampleTime
      settings: AttributesFormatString=%<Value>
  Constant7 : Constant  OutDataTypeStr=uint8  SampleTime=ap.apSampleTime
      settings: AttributesFormatString=%<Value>
  Constant8 : Constant  Value=4  OutDataTypeStr=uint8  SampleTime=ap.apSampleTime
      settings: AttributesFormatString=%<Value>
  Constant9 : Constant  OutDataTypeStr=uint8  SampleTime=ap.apSampleTime
      settings: AttributesFormatString=%<Value>
  Data Type Conversion{1..3,7} (4 alike) : DataTypeConversion  OutDataTypeStr=uint8
  Manual Switch{1..3,6..9,11} (8 alike) : ManualSwitch
  Manual Switch4 : ManualSwitch  CurrentSetting=0
  Manual Switch5 : ManualSwitch  CurrentSetting=0
  Pulse Generator : DiscretePulseGenerator  Period=300  PulseWidth=2  SampleTime=ap.apSampleTime
  Slider Gain : simulink/Math Operations/Slider Gain  gain=0  low=-18  high=18
  Slider Gain1 : simulink/Math Operations/Slider Gain  gain=150  low=0  high=800
  Slider Gain2 : simulink/Math Operations/Slider Gain  gain=21  low=1  high=55
  Step1 : Step  Time=10  After=5  SampleTime=ap.apSampleTime
  Step2 : Step  Time=10  Before=uavData.ic.Pos_0(3)  After=500  SampleTime=ap.apSampleTime
  Step3 : Step  Time=0.01  Before=1  After=0  SampleTime=ap.apSampleTime
  Step4 : Step  Time=175  Before=2  After=3  SampleTime=ap.apSampleTime
  Step5 : Step  Time=350  SampleTime=ap.apSampleTime
  Step6 : Step  Time=220  Before=18  After=21  SampleTime=ap.apSampleTime
  gsCommands : Outport  OutDataTypeStr=Bus: gsCommandsBus  VectorParamsAs1DForOutWhenUnconnected=off
  wires:
  Step6/1 -> Manual Switch5/2
  Slider Gain2/1 -> Manual Switch5/1  "U_c"
  Manual Switch5/1 -> Bus Creator/1  "U_c"
  Manual Switch4/1 -> Manual Switch7/1
  Constant6/1 -> Manual Switch4/1
  Step5/1 -> Data Type Conversion3/1
  Data Type Conversion3/1 -> Manual Switch4/2
  Compute Mobile Location/1(Mobile Location) -> Bus Creator/9  "MobileLocation"
  Manual Switch7/1 -> Bus Creator/4  "RTB"
  Constant9/1 -> Manual Switch7/2
  Bus Creator/1 -> gsCommands/1
  Constant2/1 -> Slider Gain2/1
  Constant1/1 -> Slider Gain1/1
  Slider Gain1/1 -> Manual Switch8/1
  Step2/1 -> Manual Switch8/2
  Manual Switch8/1 -> Bus Creator/2  "h_c_midLevel"
  Constant3/1 -> Slider Gain/1
  Manual Switch6/1 -> Angular Velocity Conversion/1
  Slider Gain/1 -> Manual Switch6/2
  Step1/1 -> Manual Switch6/1
  Angular Velocity Conversion/1 -> Bus Creator/3  "psiDot_c_midLevel"
  Constant4/1 -> Manual Switch1/1
  Constant5/1 -> Manual Switch1/2
  Manual Switch1/1 -> Bus Creator/5  "followMobile"
  Data Type Conversion1/1 -> Manual Switch2/1
  Constant7/1 -> Manual Switch2/2
  Manual Switch2/1 -> Bus Creator/6  "isManualModeOn"
  Constant32/1 -> Manual Switch11/2
  Constant42/1 -> Manual Switch11/1
  Step3/1 -> Data Type Conversion1/1
  Manual Switch3/1 -> Bus Creator/7  "guidanceMode"
  Step4/1 -> Data Type Conversion2/1
  Data Type Conversion2/1 -> Manual Switch3/2
  Manual Switch11/1 -> Manual Switch3/1
  Constant8/1 -> Bus Creator/8  "viewPointIdx"
  Data Type Conversion7/1 -> Manual Switch9/1
  Pulse Generator/1 -> Data Type Conversion7/1
  Constant10/1 -> Manual Switch9/2
  Manual Switch9/1 -> Bus Creator/10  "heartbeat"

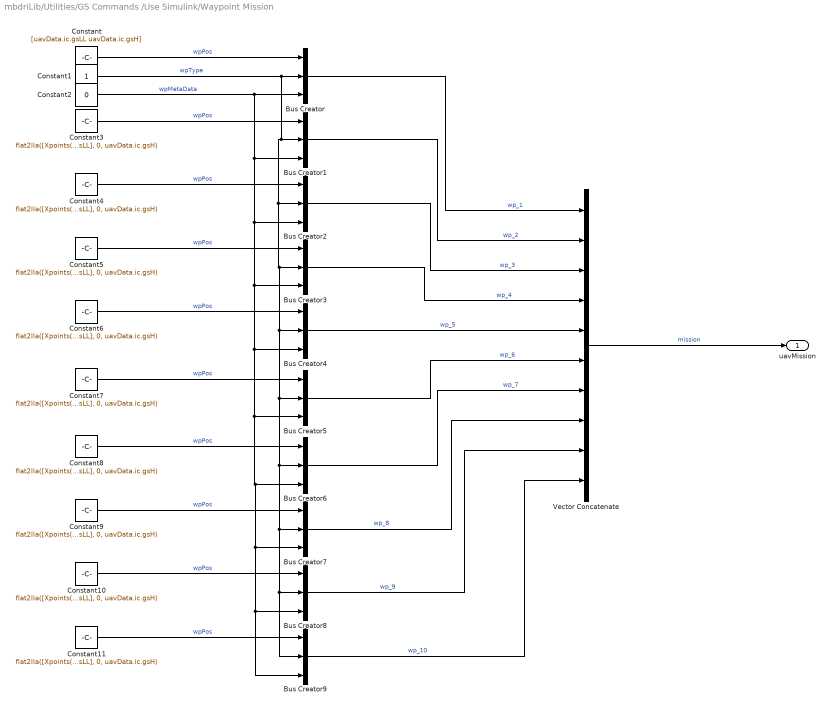
== system mbdriLib/Utilities/GS Commands /Use Simulink/Waypoint Mission ==
  Bus Creator{,1..9} (10 alike) : BusCreator  Inputs=3  OutDataTypeStr=Bus: waypoint  NonVirtualBus=on
  Constant : Constant  Value=[uavData.ic.gsLL uavData.ic.gsH]
      settings: AttributesFormatString=%<Value>
  Constant1 : Constant  OutDataTypeStr=uint8
      settings: AttributesFormatString=%<Value>
  Constant10 : Constant  Value=flat2lla([Xpoints(8) Ypoints(8) Zpoints(8)], [uavData.ic.gsLL], 0, uavData.ic.gsH)
      settings: AttributesFormatString=%<Value>
  Constant11 : Constant  Value=flat2lla([Xpoints(9) Ypoints(9) Zpoints(9)], [uavData.ic.gsLL], 0, uavData.ic.gsH)
      settings: AttributesFormatString=%<Value>
  Constant2 : Constant  Value=0
      settings: AttributesFormatString=%<Value>
  Constant3 : Constant  Value=flat2lla([Xpoints(1) Ypoints(1) Zpoints(1)], [uavData.ic.gsLL], 0, uavData.ic.gsH)
      settings: AttributesFormatString=%<Value>
  Constant4 : Constant  Value=flat2lla([Xpoints(2) Ypoints(2) Zpoints(2)], [uavData.ic.gsLL], 0, uavData.ic.gsH)
      settings: AttributesFormatString=%<Value>
  Constant5 : Constant  Value=flat2lla([Xpoints(3) Ypoints(3) Zpoints(3)], [uavData.ic.gsLL], 0, uavData.ic.gsH)
      settings: AttributesFormatString=%<Value>
  Constant6 : Constant  Value=flat2lla([Xpoints(4) Ypoints(4) Zpoints(4)], [uavData.ic.gsLL], 0, uavData.ic.gsH)
      settings: AttributesFormatString=%<Value>
  Constant7 : Constant  Value=flat2lla([Xpoints(5) Ypoints(5) Zpoints(5)], [uavData.ic.gsLL], 0, uavData.ic.gsH)
      settings: AttributesFormatString=%<Value>
  Constant8 : Constant  Value=flat2lla([Xpoints(6) Ypoints(6) Zpoints(6)], [uavData.ic.gsLL], 0, uavData.ic.gsH)
      settings: AttributesFormatString=%<Value>
  Constant9 : Constant  Value=flat2lla([Xpoints(7) Ypoints(7) Zpoints(7)], [uavData.ic.gsLL], 0, uavData.ic.gsH)
      settings: AttributesFormatString=%<Value>
  Vector Concatenate : Concatenate  NumInputs=10
  uavMission : Outport  VectorParamsAs1DForOutWhenUnconnected=off
  wires:
  Constant11/1 -> Bus Creator9/1  "wpPos"
  Bus Creator9/1 -> Vector Concatenate/10  "wp_10"
  Bus Creator8/1 -> Vector Concatenate/9  "wp_9"
  Constant10/1 -> Bus Creator8/1  "wpPos"
  Constant9/1 -> Bus Creator7/1  "wpPos"
  Bus Creator7/1 -> Vector Concatenate/8  "wp_8"
  Vector Concatenate/1 -> uavMission/1  "mission"
  Constant/1 -> Bus Creator/1  "wpPos"
  Bus Creator/1 -> Vector Concatenate/1  "wp_1"
  Bus Creator1/1 -> Vector Concatenate/2  "wp_2"
  Bus Creator2/1 -> Vector Concatenate/3  "wp_3"
  Bus Creator3/1 -> Vector Concatenate/4  "wp_4"
  Bus Creator4/1 -> Vector Concatenate/5  "wp_5"
  Bus Creator5/1 -> Vector Concatenate/6  "wp_6"
  Bus Creator6/1 -> Vector Concatenate/7  "wp_7"
  Constant3/1 -> Bus Creator1/1  "wpPos"
  Constant4/1 -> Bus Creator2/1  "wpPos"
  Constant5/1 -> Bus Creator3/1  "wpPos"
  Constant6/1 -> Bus Creator4/1  "wpPos"
  Constant7/1 -> Bus Creator5/1  "wpPos"
  Constant8/1 -> Bus Creator6/1  "wpPos"
  Constant1/1 -> Bus Creator2/2, Bus Creator3/2, Bus Creator4/2, Bus Creator6/2, Bus Creator7/2, Bus Creator8/2, Bus Creator9/2, Bus Creator5/2, Bus Creator1/2, Bus Creator/2  "wpType"
  Constant2/1 -> Bus Creator2/3, Bus Creator3/3, Bus Creator4/3, Bus Creator6/3, Bus Creator7/3, Bus Creator8/3, Bus Creator9/3, Bus Creator5/3, Bus Creator1/3, Bus Creator/3  "wpMetaData"

== system mbdriLib/Utilities/GS Commands /Use Simulink/Ground Station Commands/Compute Mobile Location ==
  note: Simple 2D Car Motion Model
  Car Model Input Profiles : SignalEditorBlockLib/Signal Editor  FileName=carModelInputProfiles.mat  ActiveScenario=High_Speed  ActiveSignal=Heading (Deg)  IsBus=off  OutputBusObjectStr=Bus: BusObject  SampleTime=ap.apSampleTime  Interpolate=off  ZeroCross=off  OutputAfterFinalValue=Setting to zero  Unit=inherit  PreserveSignalName=on
  Constant : Constant  Value=uavData.ic.gsH
      settings: AttributesFormatString=%<Value>
  Flat Earth to LLA : aerolibtransform2/Flat Earth to LLA  units=Metric (MKS)  ptype=Earth (WGS84)  F=1/298.257223563  R=6378137  refPosPort=off  LL0=uavData.ic.gsLL  psi=0
  Mux : Mux  Inputs=2
  Simple Car Model : Subsystem
  Mobile Location : Outport  VectorParamsAs1DForOutWhenUnconnected=off
  wires:
  Flat Earth to LLA/2 -> Mux/2
  Simple Car Model/1(basePoint) -> Flat Earth to LLA/1
  Mux/1 -> Mobile Location/1  "MobileLocation"
  Constant/1 -> Flat Earth to LLA/2
  Car Model Input Profiles/2 -> Simple Car Model/2(Speed)
  Flat Earth to LLA/1 -> Mux/1
  Car Model Input Profiles/1 -> Simple Car Model/1(Heading)

== system mbdriLib/Utilities/GS Commands /Use Simulink/Ground Station Commands/Compute Mobile Location/Simple Car Model ==
  Heading : Inport
  Speed : Inport  Port=2
  Heading/Speed to Velocity : Subsystem
  Simple Car Model : Subsystem
  basePoint : Outport  VectorParamsAs1DForOutWhenUnconnected=off
  wires:
  Heading/Speed to Velocity/1(Velocity) -> Simple Car Model/1(Velocity)
  Heading/1 -> Heading/Speed to Velocity/1(Heading)
  Simple Car Model/1(p_cg) -> basePoint/1
  Speed/1 -> Heading/Speed to Velocity/2(Speed)

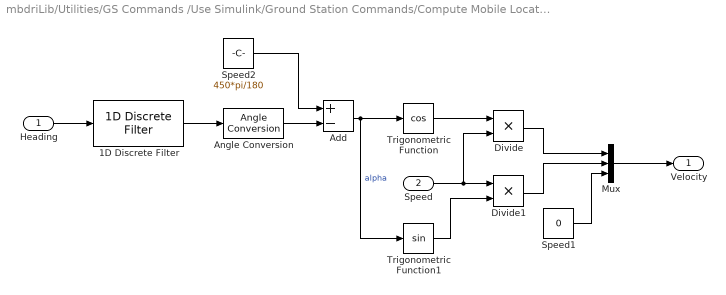
== system mbdriLib/Utilities/GS Commands /Use Simulink/Ground Station Commands/Compute Mobile Location/Simple Car Model/Heading//Speed to Velocity ==
  Heading : Inport
  Speed : Inport  Port=2
  1D Discrete Filter : $bdroot/Filtering/1D Discrete Filter  bw=10  TSample=ap.apSampleTime
      settings: AttributesFormatString=Fc = 10
  Add : Sum  Inputs=+-
  Angle Conversion : aerolibconvert2/Angle Conversion  IU=deg  OU=rad
  Divide : Product
  Divide1 : Product
  Mux : Mux  Inputs=3
  Speed1 : Constant  Value=0  SampleTime=ap.apSampleTime
      settings: AttributesFormatString=%<Value>
  Speed2 : Constant  Value=450*pi/180  SampleTime=ap.apSampleTime
      settings: AttributesFormatString=%<Value>
  Trigonometric Function : Trigonometry  Operator=cos
  Trigonometric Function1 : Trigonometry
  Velocity : Outport  VectorParamsAs1DForOutWhenUnconnected=off
  wires:
  Speed1/1 -> Mux/3
  Speed2/1 -> Add/1
  Add/1 -> Trigonometric Function/1, Trigonometric Function1/1  "alpha"
  Trigonometric Function/1 -> Divide/1
  Divide/1 -> Mux/1
  Angle Conversion/1 -> Add/2
  Divide1/1 -> Mux/2
  Trigonometric Function1/1 -> Divide1/2
  1D Discrete Filter/1 -> Angle Conversion/1
  Mux/1 -> Velocity/1
  Heading/1 -> 1D Discrete Filter/1
  Speed/1 -> Divide1/1, Divide/2

== system mbdriLib/Utilities/GS Commands /Use Simulink/Ground Station Commands/Compute Mobile Location/Simple Car Model/Simple Car Model ==
  Velocity : Inport
  Constant13 : Constant  Value=[0 0 0]  SampleTime=ap.apSampleTime
      settings: AttributesFormatString=%<Value>
  Discrete-Time Integrator : DiscreteIntegrator  InitialConditionSource=external  SampleTime=-1  ICPrevOutput=DiscIntNeverNeededParam  ICPrevScaledInput=DiscIntNeverNeededParam
  p_cg : Outport  VectorParamsAs1DForOutWhenUnconnected=off
  wires:
  Constant13/1 -> Discrete-Time Integrator/2
  Discrete-Time Integrator/1 -> p_cg/1
  Velocity/1 -> Discrete-Time Integrator/1

== stateflow chart mbdriLib/Guidance/Wp Switching Logic ==
  state TO_IP
    entry:
    toWp = uint8(2);
    fromWp = uint8(1);
  state REACHED_IP
    state SWITCH_WP
      entry:
      fromWp = toWp;
      if (toWp +1 <= MaxWp)
      toWp = toWp + 1;
      else
      toWp = uint8(2);
      end
    state FLYING
    (default) -> SWITCH_WP
    SWITCH_WP -> FLYING
    FLYING -> SWITCH_WP : [distance_to_switch <= 0]
  (default) -> TO_IP
  REACHED_IP -> TO_IP : [wpEnable == 1]
  TO_IP -> REACHED_IP : [distance_to_switch <= 0]
  data: distance_to_switch input; fromWp output uint8; toWp output uint8; MaxWp input uint8; wpEnable input
